simulink model "ED_Project_2"  (R2021b)
settings: Solver=VariableStepAuto  StartTime=0.0  StopTime=1  RelTol=1e-3
libraries: spsThyristorLib x12, spsSeriesRLCBranchLib x2, spsSynchronousMachineSIFundamentalLib x1, spsThreePhaseSourceLib x1, spspowerguiLib x1
settings Model: Creator=student  LastModifiedBy=student

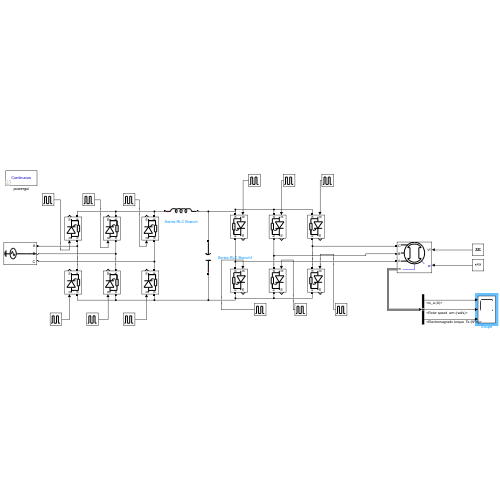
[thumbnail: Simulink's stored preview of the top-level diagram]
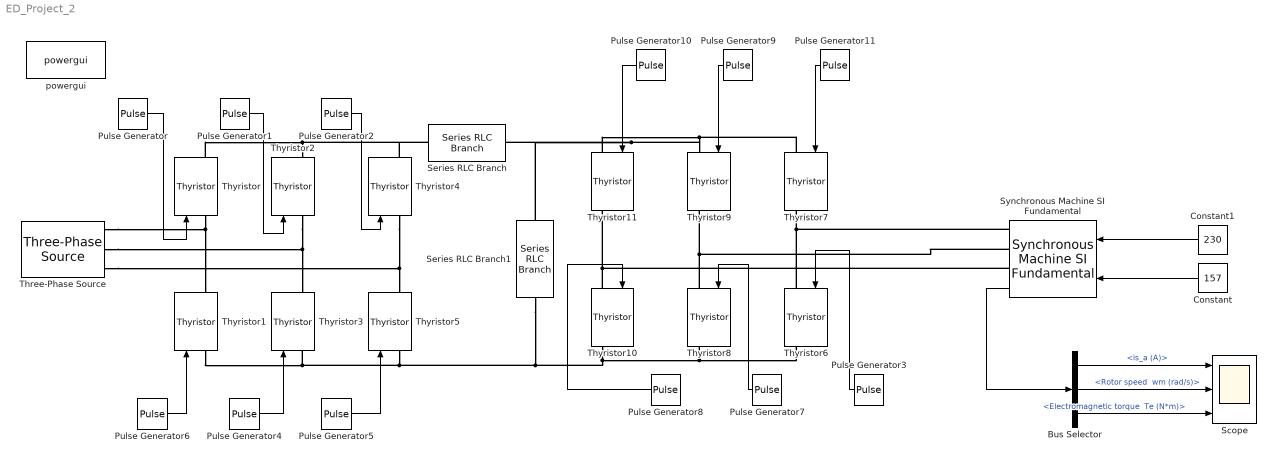
== system ED_Project_2 ==
  Bus Selector : BusSelector  OutputSignals="Stator current.is_a (A),Mechanical.Rotor speed  wm (rad/s),Mechanical.Electromagnetic torque  Te (N*m)"
  Constant : Constant  Value=157
  Constant1 : Constant  Value=230
  Pulse Generator : DiscretePulseGenerator  PulseType=Time based  Period=1/50  PulseWidth=30
  Pulse Generator1 : DiscretePulseGenerator  PulseType=Time based  Period=1/50  PulseWidth=30  PhaseDelay=0.0066
  Pulse Generator10 : DiscretePulseGenerator  PulseType=Time based  Period=1/50  PulseWidth=30  PhaseDelay=0.0233
  Pulse Generator11 : DiscretePulseGenerator  PulseType=Time based  Period=1/50  PulseWidth=30  PhaseDelay=0.01
  Pulse Generator2 : DiscretePulseGenerator  PulseType=Time based  Period=1/50  PulseWidth=30  PhaseDelay=0.013
  Pulse Generator3 : DiscretePulseGenerator  PulseType=Time based  Period=1/50  PulseWidth=30
  Pulse Generator4 : DiscretePulseGenerator  PulseType=Time based  Period=1/50  PulseWidth=30  PhaseDelay=0.0166
  Pulse Generator5 : DiscretePulseGenerator  PulseType=Time based  Period=1/50  PulseWidth=30  PhaseDelay=0.0233
  Pulse Generator6 : DiscretePulseGenerator  PulseType=Time based  Period=1/50  PulseWidth=30  PhaseDelay=0.01
  Pulse Generator7 : DiscretePulseGenerator  PulseType=Time based  Period=1/50  PulseWidth=30  PhaseDelay=0.0066
  Pulse Generator8 : DiscretePulseGenerator  PulseType=Time based  Period=1/50  PulseWidth=30  PhaseDelay=0.013
  Pulse Generator9 : DiscretePulseGenerator  PulseType=Time based  Period=1/50  PulseWidth=30  PhaseDelay=0.0166
  Scope : Scope  NumInputPorts=3
  Series RLC Branch : spsSeriesRLCBranchLib/Series RLC Branch  LConnTagsString=__new0  RConnTagsString=__new0  BranchType=L  Resistance=100  Inductance=1e-3  SetiL0=off  InitialCurrent=0  Capacitance=1e-6  Setx0=off  InitialVoltage=0  Measurements=None
  Series RLC Branch1 : spsSeriesRLCBranchLib/Series RLC Branch  LConnTagsString=__new0  RConnTagsString=__new0  BranchType=C  Resistance=100  Inductance=1e-3  SetiL0=off  InitialCurrent=0  Capacitance=1e-6  Setx0=off  InitialVoltage=0  Measurements=None
  Synchronous Machine SI Fundamental : spsSynchronousMachineSIFundamentalLib/Synchronous Machine SI Fundamental  PresetModel=01: 50Hz 400V 8.1kVA 1500RPM  MechanicalLoad=Speed w  ShowDetailedParameters=on  RotorType=Salient-pole  Units=SI fundamental parameters  MeasurementBus=off  NominalParameters=[8100 400 50]  Stator=[1.62 0.004527 0.1086 0.05175]  Field=[1.208 0.01132]  Dampers2=[ 0.0664, 1.387e-3, 0.0292, 6.896e-4, 7.907e-3, 2.477e-3]  Dampers1=[3.142 0.007334 4.772 0.01015]  Mechanical=[0.0923 0.009 2]  PolePairs=2  InitialConditions="[ 0  0  0  0  0  0  0  0  70.3192 ]"  SetSaturation=off  Saturation=[695.64,774.7,917.5,1001.6,1082.2,1175.9,1293.6,1430.2,1583.7;9660,10623,12243,13063,13757,14437,15180,15890,16567]  DisplayVfd=off  LoadFlowParameters=[1,0,0,0,0]  TsPowergui=0  TsBlock=-1  IterativeModel=Trapezoidal non iterative  IterativeDiscreteModel=Trapezoidal non iterative  BusType=PV  Pref=0  Qref=0  Qmin=-inf  Qmax=inf  PLF=0  QLF=0
      settings: SourceProductBaseCode=PS
  Three-Phase Source : spsThreePhaseSourceLib/Three-Phase Source  InternalConnection=Yg  VoltagePhases=off  Voltage=415  PhaseAngle=0  Voltage_phases=[25e3 25e3 25e3]/sqrt(3)  PhaseAngles_phases=[0 -120 +120]  Frequency=50  NonIdealSource=off  SpecifyImpedance=off  Resistance=0.8929  Inductance=16.58e-3  ShortCircuitLevel=100e6  BaseVoltage=25e3  XRratio=7  BusType=swing  Pref=10e3  Qref=0  Prefabc=[10e3, 10e3, 10e3]  Qrefabc=[0, 0, 0]  Qmin=-inf  Qmax=inf
  Thyristor{,1..11} (12 alike) : spsThyristorLib/Thyristor  Ron=0.001  Lon=0  Vf=0.8  IC=0  Rs=500  Cs=250e-9  Measurements=on
  powergui : spspowerguiLib/powergui  Priority=1  SimulationMode=Continuous  SampleTime=50e-6  frequency=60  Iterations=50  frequencyindice=0  Pbase=100e6  ErrMax=1e-4  UnitsV=kV  UnitsW=MW  buscounter=0  FunctionMessages=off  echomessages=off  EnableUseOfTLC=off  CurrentSourceSwitches=off  DisableSnubberDevices=off  DisableRonSwitches=off  DisableVfSwitches=off  DisplayEquations=off  AutomaticDiscreteSolvers=off  SolverType=Tustin/Backward Euler (TBE)  Interpol=off  ExternalGateDelay=off  methode=off  Ts=100  x0status=blocks  SPID=on  SwTol=0  HookPort=off  NonlinearTolerance=1e-4  nMaxIteration=100  ContinueOnMaxIteration=off  RestoreLinks=warning  ResistiveCurrentMeasurement=off  Frange=[0:2:500]  Ylog=off  Xlog=on  ShowGrid=off  save=off  variable=ZData  structure=0  ZoomFFT=off  StartTime=0.0  cycles=1  DisplayStyle=1  fundamental=60  FreqAxis=off  MaxFrequency=1000  frequencyindicesteady=1  RmsSteady=1  display=off
  wires:
  Pulse Generator/1 -> Thyristor/1
  Pulse Generator1/1 -> Thyristor2/1
  Pulse Generator2/1 -> Thyristor4/1
  Pulse Generator6/1 -> Thyristor1/1
  Pulse Generator4/1 -> Thyristor3/1
  Pulse Generator5/1 -> Thyristor5/1
  Pulse Generator3/1 -> Thyristor6/1
  Pulse Generator11/1 -> Thyristor7/1
  Pulse Generator8/1 -> Thyristor10/1
  Pulse Generator7/1 -> Thyristor8/1
  Pulse Generator10/1 -> Thyristor11/1
  Pulse Generator9/1 -> Thyristor9/1
  Constant/1 -> Synchronous Machine SI Fundamental/1
  Synchronous Machine SI Fundamental/1 -> Bus Selector/1
  Bus Selector/1 -> Scope/1  "<is_a (A)>"
  Bus Selector/2 -> Scope/2  "<Rotor speed  wm (rad/s)>"
  Bus Selector/3 -> Scope/3  "<Electromagnetic torque  Te (N*m)>"
  Constant1/1 -> Synchronous Machine SI Fundamental/2
  connections:
  Thyristor/LConn1 -- Thyristor1/RConn1 -- Three-Phase Source/RConn1
  Thyristor2/LConn1 -- Three-Phase Source/RConn2 -- Thyristor3/RConn1
  Thyristor4/LConn1 -- Three-Phase Source/RConn3 -- Thyristor5/RConn1
  Thyristor10/RConn1 -- Thyristor1/LConn1 -- Thyristor3/LConn1 -- Thyristor5/LConn1 -- Series RLC Branch1/LConn1 -- Thyristor6/RConn1 -- Thyristor8/RConn1
  Thyristor/RConn1 -- Series RLC Branch/LConn1 -- Thyristor4/RConn1 -- Thyristor2/RConn1
  Thyristor9/LConn1 -- Series RLC Branch/RConn1 -- Series RLC Branch1/RConn1 -- Thyristor11/LConn1 -- Thyristor7/LConn1
  Thyristor6/LConn1 -- Synchronous Machine SI Fundamental/RConn3 -- Thyristor7/RConn1
  Thyristor8/LConn1 -- Synchronous Machine SI Fundamental/RConn2 -- Thyristor9/RConn1
  Thyristor10/LConn1 -- Thyristor11/RConn1 -- Synchronous Machine SI Fundamental/RConn1
